simulink model "shahidspwmthreephase"  (Simulink 7.5)
settings: Solver=ode45  StartTime=0.0  StopTime=3  RelTol=1e-3
libraries: powerlib x11, powerlib_extras x6
settings Model: Creator=SHAHID  LastModifiedBy=SHAHID

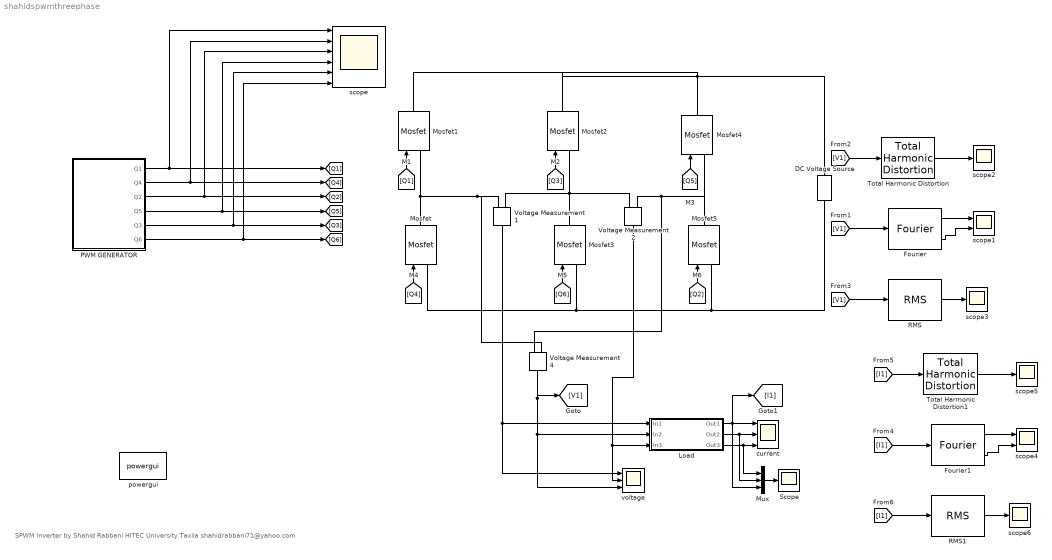
== system shahidspwmthreephase ==
  note: SPWM Inverter by Shahid Rabbani
      | HITEC University Taxila
      | shahidrabbani71@yahoo.com
  " current" : Scope  NumInputPorts=3
      settings: YMin=-0.7~-0.8~-0.7  YMax=0.8~0.7~0.7
  DC Voltage Source : powerlib/Electrical Sources/DC Voltage Source  DialogController=POWERSYS.PowerSysDialog  SystemSampleTime=-1  Amplitude=400  Measurements=Voltage
  Fourier : powerlib_extras/Measurements/Fourier  DialogController=POWERSYS.PowerSysDialog  SystemSampleTime=-1  f1=50  n=3
  Fourier1 : powerlib_extras/Measurements/Fourier  DialogController=POWERSYS.PowerSysDialog  SystemSampleTime=-1  f1=50  n=3
  Load : Subsystem
  Mosfet{,1..5} (6 alike) : powerlib/Power Electronics/Mosfet  DialogController=POWERSYS.PowerSysDialog  SystemSampleTime=-1  Ron=0.01  Lon=0  Rd=0.01  Vfd=0  IC=0  Rs=1e5  Cs=inf  Measurements=off
  Mux : Mux  Inputs=3
  PWM GENERATOR : Subsystem
  RMS : powerlib_extras/Measurements/RMS  DialogController=POWERSYS.PowerSysDialog  SystemSampleTime=-1  f1=50
  RMS1 : powerlib_extras/Measurements/RMS  DialogController=POWERSYS.PowerSysDialog  SystemSampleTime=-1  f1=50
  Scope : Scope
      settings: YMin=-1  YMax=1.2  SaveName=ScopeData2
  Total Harmonic Distortion : powerlib_extras/Measurements/Total Harmonic Distortion  DialogController=POWERSYS.PowerSysDialog  SystemSampleTime=-1  f1=50
  Total Harmonic Distortion1 : powerlib_extras/Measurements/Total Harmonic Distortion  DialogController=POWERSYS.PowerSysDialog  SystemSampleTime=-1  f1=50
  Voltage Measurement1 : powerlib/Measurements/Voltage Measurement  DialogController=POWERSYS.PowerSysDialog  SystemSampleTime=-1  PhasorSimulation=off  OutputType=Complex  PSBequivalent=0
  Voltage Measurement2 : powerlib/Measurements/Voltage Measurement  DialogController=POWERSYS.PowerSysDialog  SystemSampleTime=-1  PhasorSimulation=off  OutputType=Complex  PSBequivalent=0
  Voltage Measurement4 : powerlib/Measurements/Voltage Measurement  DialogController=POWERSYS.PowerSysDialog  SystemSampleTime=-1  PhasorSimulation=off  OutputType=Complex  PSBequivalent=0
  powergui : powerlib/powergui  Priority=1  SystemSampleTime=-1  SimulationMode=Continuous  SampleTime=50e-6  frequency=60  SPID=off  DisableSnubberDevices=off  DisableRonSwitches=off  DisableVfSwitches=off  SwTol=0  Interpol=off  frequencyindice=0  echomessages=off  HookPort=off  DisplayEquations=off  FunctionMessages=off  EnableUseOfTLC=off  x0status=blocks  RestoreLinks=warning  ResistiveCurrentMeasurement=off  Ylog=off  Xlog=on  ShowGrid=off  save=off  variable=ZData  ZoomFFT=off  StartTime=0.0  cycles=1  DisplayStyle=1  FreqAxis=off  MaxFrequency=1000  frequencyindicesteady=1  display=off  methode=off
  scope : Scope  NumInputPorts=6
      settings: YMin=0~0~0~0~0~0  YMax=1~1~1~1~1~1
  scope1 : Scope  NumInputPorts=2
      settings: YMin=-0.8~-150  YMax=0.8~150  SaveName=ScopeData3
  scope{2..3,5..6} (4 alike) : Scope
      scope2 settings: YMin=-1  YMax=1  SaveName=ScopeData4
      scope3 settings: YMin=72.241  YMax=72.241  SaveName=ScopeData5
      scope5 settings: YMin=-1  YMax=1  SaveName=ScopeData8
      scope6 settings: YMin=68.629  YMax=75.853  SaveName=ScopeData9
  scope4 : Scope  NumInputPorts=2
      settings: YMin=-0.8~-150  YMax=0.8~150  SaveName=ScopeData7
  "voltage " : Scope  NumInputPorts=3
      settings: YMin=-150~-1~-5  YMax=150~1~5  SaveName=ScopeData6
  wires:
  [Q3] -> Mosfet2/1
  [Q1] -> Mosfet1/1
  Fourier/1 -> scope1/1
  Fourier/2 -> scope1/2
  [V1] -> Fourier/1
  Total Harmonic Distortion/1 -> scope2/1
  [V1] -> Total Harmonic Distortion/1
  RMS/1 -> scope3/1
  [V1] -> RMS/1
  [Q5] -> Mosfet4/1
  [Q4] -> Mosfet/1
  [Q6] -> Mosfet3/1
  [Q2] -> Mosfet5/1
  PWM GENERATOR/1(Q1) -> [Q1], scope/1
  PWM GENERATOR/2(Q4) -> [Q4], scope/2
  PWM GENERATOR/3(Q2) -> [Q2], scope/3
  PWM GENERATOR/4(Q5) -> [Q5], scope/4
  PWM GENERATOR/5(Q3) -> [Q3], scope/5
  PWM GENERATOR/6(Q6) -> [Q6], scope/6
  Voltage Measurement1/1 -> "voltage "/1, Load/1(In1)
  Voltage Measurement2/1 -> "voltage "/2, Load/3(In3)
  Voltage Measurement4/1 -> "voltage "/3, Load/2(In2), [V1]
  Load/1(Out1) -> " current"/1, Mux/3, [I1]
  Load/2(Out2) -> " current"/2, Mux/2
  Load/3(Out3) -> " current"/3, Mux/1
  Mux/1 -> Scope/1
  Fourier1/1 -> scope4/1
  Fourier1/2 -> scope4/2
  [I1] -> Fourier1/1
  Total Harmonic Distortion1/1 -> scope5/1
  [I1] -> Total Harmonic Distortion1/1
  RMS1/1 -> scope6/1
  [I1] -> RMS1/1
  connections:
  Mosfet1/RConn1 -- Mosfet2/RConn1 -- Mosfet4/RConn1 -- DC Voltage Source/RConn1
  Mosfet3/RConn1 -- Mosfet2/LConn1 -- Voltage Measurement1/LConn2 -- Voltage Measurement2/LConn1
  Voltage Measurement1/LConn1 -- Mosfet1/LConn1 -- Mosfet/RConn1 -- Voltage Measurement4/LConn2
  Mosfet5/LConn1 -- Mosfet3/LConn1 -- Mosfet/LConn1 -- DC Voltage Source/LConn1
  Mosfet5/RConn1 -- Mosfet4/LConn1 -- Voltage Measurement2/LConn2 -- Voltage Measurement4/LConn1

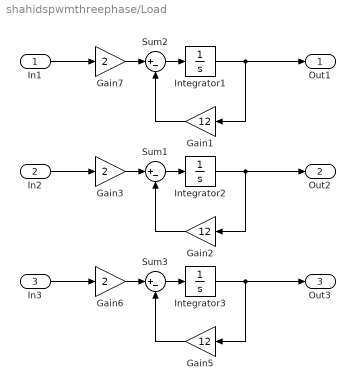
== system shahidspwmthreephase/Load ==
  In1 : Inport  OutDataType=fixdt(1, 16)  OutScaling=2^0
  In2 : Inport  Port=2  OutDataType=fixdt(1, 16)  OutScaling=2^0
  In3 : Inport  Port=3  OutDataType=fixdt(1, 16)  OutScaling=2^0
  Gain1 : Gain  Gain=12  ParameterDataType=fixdt(1, 16)  ParameterScaling=2^0  OutDataType=fixdt(1, 16)  OutScaling=2^0
  Gain2 : Gain  Gain=12  ParameterDataType=fixdt(1, 16)  ParameterScaling=2^0  OutDataType=fixdt(1, 16)  OutScaling=2^0
  Gain3 : Gain  Gain=2  ParameterDataType=fixdt(1, 16)  ParameterScaling=2^0  OutDataType=fixdt(1, 16)  OutScaling=2^0
  Gain5 : Gain  Gain=12  ParameterDataType=fixdt(1, 16)  ParameterScaling=2^0  OutDataType=fixdt(1, 16)  OutScaling=2^0
  Gain6 : Gain  Gain=2  ParameterDataType=fixdt(1, 16)  ParameterScaling=2^0  OutDataType=fixdt(1, 16)  OutScaling=2^0
  Gain7 : Gain  Gain=2  ParameterDataType=fixdt(1, 16)  ParameterScaling=2^0  OutDataType=fixdt(1, 16)  OutScaling=2^0
  Integrator1 : Integrator
  Integrator2 : Integrator
  Integrator3 : Integrator
  Sum1 : Sum  Inputs=|+-  OutDataType=fixdt(1, 16)  OutScaling=2^0
  Sum2 : Sum  Inputs=|+-  OutDataType=fixdt(1, 16)  OutScaling=2^0
  Sum3 : Sum  Inputs=|+-  OutDataType=fixdt(1, 16)  OutScaling=2^0
  Out1 : Outport  OutDataType=fixdt(1, 16)  OutScaling=2^0
  Out2 : Outport  Port=2  OutDataType=fixdt(1, 16)  OutScaling=2^0
  Out3 : Outport  Port=3  OutDataType=fixdt(1, 16)  OutScaling=2^0
  wires:
  Integrator1/1 -> Gain1/1, Out1/1
  Gain7/1 -> Sum2/1
  Sum2/1 -> Integrator1/1
  Gain1/1 -> Sum2/2
  In1/1 -> Gain7/1
  Integrator2/1 -> Gain2/1, Out2/1
  Gain3/1 -> Sum1/1
  Sum1/1 -> Integrator2/1
  Gain2/1 -> Sum1/2
  In2/1 -> Gain3/1
  Integrator3/1 -> Gain5/1, Out3/1
  Gain6/1 -> Sum3/1
  Sum3/1 -> Integrator3/1
  Gain5/1 -> Sum3/2
  In3/1 -> Gain6/1

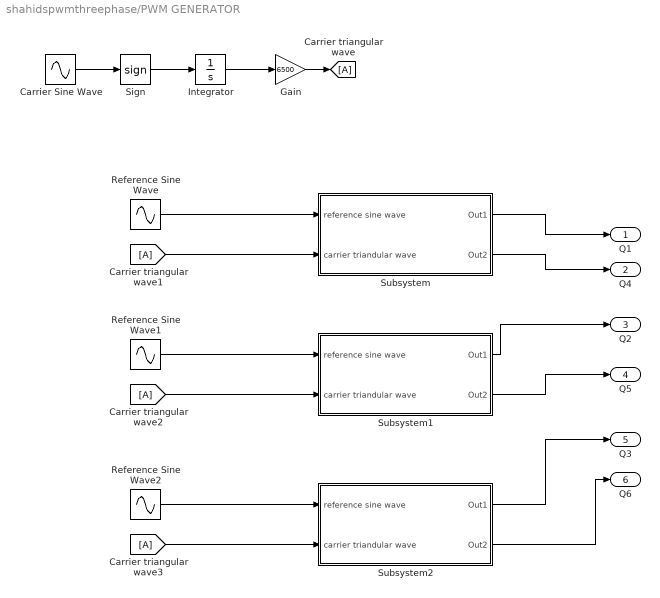
== system shahidspwmthreephase/PWM GENERATOR ==
  Carrier Sine Wave : Sin  Amplitude=1  Bias=0  Frequency=2*pi*3000  Phase=0  Samples=10  SampleTime=0  Offset=0
  Gain : Gain  Gain=6500  ParameterDataType=fixdt(1, 16)  ParameterScaling=2^0  OutDataType=fixdt(1, 16)  OutScaling=2^0
  Integrator : Integrator
  Reference Sine Wave : Sin  Amplitude=1  Bias=0  Frequency=2*pi*50  Phase=0  Samples=10  SampleTime=0  Offset=0
  Reference Sine Wave1 : Sin  Amplitude=1  Bias=0  Frequency=2*pi*50  Phase=-pi/3  Samples=10  SampleTime=0  Offset=0
  Reference Sine Wave2 : Sin  Amplitude=1  Bias=0  Frequency=2*pi*50  Phase=-2*pi/3  Samples=10  SampleTime=0  Offset=0
  Sign : Signum
  Subsystem : Subsystem
  Subsystem1 : Subsystem
  Subsystem2 : Subsystem
  Q1 : Outport  OutDataType=fixdt(1, 16)  OutScaling=2^0
  Q4 : Outport  Port=2  OutDataType=fixdt(1, 16)  OutScaling=2^0
  Q2 : Outport  Port=3  OutDataType=fixdt(1, 16)  OutScaling=2^0
  Q5 : Outport  Port=4  OutDataType=fixdt(1, 16)  OutScaling=2^0
  Q3 : Outport  Port=5  OutDataType=fixdt(1, 16)  OutScaling=2^0
  Q6 : Outport  Port=6  OutDataType=fixdt(1, 16)  OutScaling=2^0
  wires:
  Carrier Sine Wave/1 -> Sign/1
  Sign/1 -> Integrator/1
  Integrator/1 -> Gain/1
  Gain/1 -> [A]
  Reference Sine Wave/1 -> Subsystem/1(reference sine wave)
  Reference Sine Wave1/1 -> Subsystem1/1(reference sine wave)
  Reference Sine Wave2/1 -> Subsystem2/1(reference sine wave)
  [A] -> Subsystem/2(carrier triandular wave)
  [A] -> Subsystem2/2(carrier triandular wave)
  [A] -> Subsystem1/2(carrier triandular wave)
  Subsystem/1(Out1) -> Q1/1
  Subsystem/2(Out2) -> Q4/1
  Subsystem1/1(Out1) -> Q2/1
  Subsystem1/2(Out2) -> Q5/1
  Subsystem2/1(Out1) -> Q3/1
  Subsystem2/2(Out2) -> Q6/1

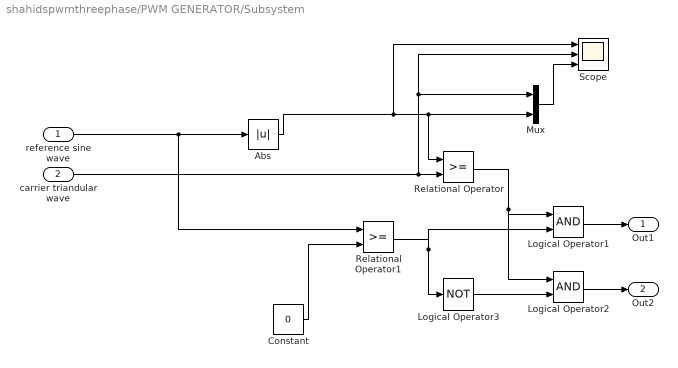
== system shahidspwmthreephase/PWM GENERATOR/Subsystem ==
  reference sine wave : Inport  OutDataType=fixdt(1, 16)  OutScaling=2^0
  carrier triandular wave : Inport  Port=2  OutDataType=fixdt(1, 16)  OutScaling=2^0
  Abs : Abs  OutDataType=fixdt(1, 16)  OutScaling=2^0
  Constant : Constant  Value=0  OutDataType=fixdt(1, 16)  OutScaling=2^0
  Logical Operator1 : Logic  AllPortsSameDT=off  OutDataTypeMode=boolean  LogicDataType=fixdt(0, 8)  OutDataTypeStr=boolean
  Logical Operator2 : Logic  AllPortsSameDT=off  OutDataTypeMode=boolean  LogicDataType=fixdt(0, 8)  OutDataTypeStr=boolean
  Logical Operator3 : Logic  Operator=NOT  AllPortsSameDT=off  OutDataTypeMode=boolean  LogicDataType=fixdt(0, 8)  OutDataTypeStr=boolean
  Mux : Mux  Inputs=2
  Relational Operator : RelationalOperator  LogicDataType=fixdt(1,16)  InputSameDT=on
  Relational Operator1 : RelationalOperator  LogicDataType=fixdt(1,16)  InputSameDT=on
  Scope : Scope  NumInputPorts=3
      settings: TickLabels=on  TimeRange=3  YMin=5.55112e-017~-0.1~-0.1  YMax=1~1.1~1.1  SaveName=ScopeData10
  Out1 : Outport  OutDataType=fixdt(1, 16)  OutScaling=2^0
  Out2 : Outport  Port=2  OutDataType=fixdt(1, 16)  OutScaling=2^0
  wires:
  Abs/1 -> Scope/1, Relational Operator/1, Mux/2
  Logical Operator3/1 -> Logical Operator2/2
  Relational Operator/1 -> Logical Operator1/1, Logical Operator2/1
  Constant/1 -> Relational Operator1/2
  Relational Operator1/1 -> Logical Operator3/1, Logical Operator1/2
  Logical Operator1/1 -> Out1/1
  Logical Operator2/1 -> Out2/1
  Mux/1 -> Scope/3
  reference sine wave/1 -> Abs/1, Relational Operator1/1
  carrier triandular wave/1 -> Relational Operator/2, Scope/2, Mux/1

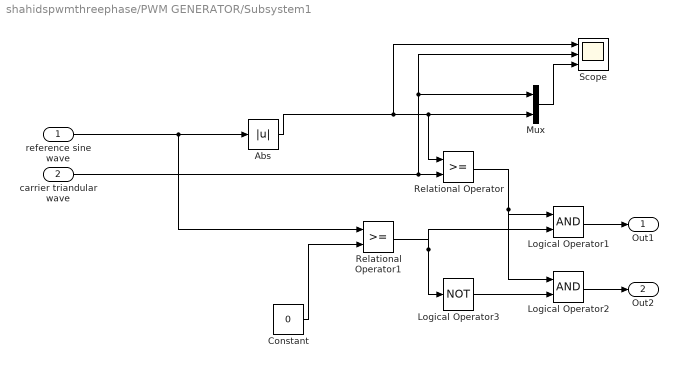
== system shahidspwmthreephase/PWM GENERATOR/Subsystem1 ==
  reference sine wave : Inport  OutDataType=fixdt(1, 16)  OutScaling=2^0
  carrier triandular wave : Inport  Port=2  OutDataType=fixdt(1, 16)  OutScaling=2^0
  Abs : Abs  OutDataType=fixdt(1, 16)  OutScaling=2^0
  Constant : Constant  Value=0  OutDataType=fixdt(1, 16)  OutScaling=2^0
  Logical Operator1 : Logic  AllPortsSameDT=off  OutDataTypeMode=boolean  LogicDataType=fixdt(0, 8)  OutDataTypeStr=boolean
  Logical Operator2 : Logic  AllPortsSameDT=off  OutDataTypeMode=boolean  LogicDataType=fixdt(0, 8)  OutDataTypeStr=boolean
  Logical Operator3 : Logic  Operator=NOT  AllPortsSameDT=off  OutDataTypeMode=boolean  LogicDataType=fixdt(0, 8)  OutDataTypeStr=boolean
  Mux : Mux  Inputs=2
  Relational Operator : RelationalOperator  LogicDataType=fixdt(1,16)  InputSameDT=on
  Relational Operator1 : RelationalOperator  LogicDataType=fixdt(1,16)  InputSameDT=on
  Scope : Scope  NumInputPorts=3
      settings: TickLabels=on  TimeRange=3  YMin=5.55112e-017~-0.1~-0.1  YMax=1~1.1~1.1  SaveName=ScopeData10
  Out1 : Outport  OutDataType=fixdt(1, 16)  OutScaling=2^0
  Out2 : Outport  Port=2  OutDataType=fixdt(1, 16)  OutScaling=2^0
  wires:
  Abs/1 -> Scope/1, Relational Operator/1, Mux/2
  Logical Operator3/1 -> Logical Operator2/2
  Relational Operator/1 -> Logical Operator1/1, Logical Operator2/1
  Constant/1 -> Relational Operator1/2
  Relational Operator1/1 -> Logical Operator3/1, Logical Operator1/2
  Logical Operator1/1 -> Out1/1
  Logical Operator2/1 -> Out2/1
  Mux/1 -> Scope/3
  reference sine wave/1 -> Abs/1, Relational Operator1/1
  carrier triandular wave/1 -> Relational Operator/2, Scope/2, Mux/1

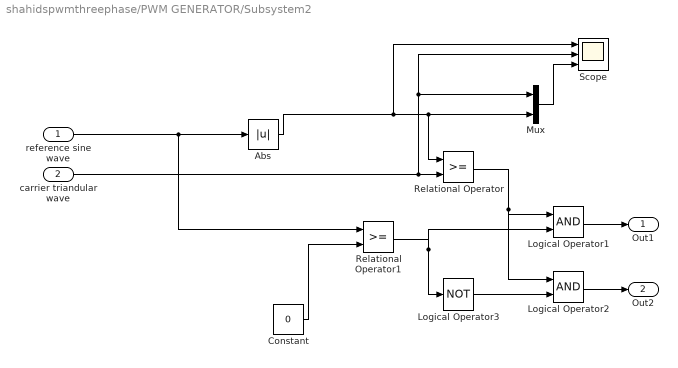
== system shahidspwmthreephase/PWM GENERATOR/Subsystem2 ==
  reference sine wave : Inport  OutDataType=fixdt(1, 16)  OutScaling=2^0
  carrier triandular wave : Inport  Port=2  OutDataType=fixdt(1, 16)  OutScaling=2^0
  Abs : Abs  OutDataType=fixdt(1, 16)  OutScaling=2^0
  Constant : Constant  Value=0  OutDataType=fixdt(1, 16)  OutScaling=2^0
  Logical Operator1 : Logic  AllPortsSameDT=off  OutDataTypeMode=boolean  LogicDataType=fixdt(0, 8)  OutDataTypeStr=boolean
  Logical Operator2 : Logic  AllPortsSameDT=off  OutDataTypeMode=boolean  LogicDataType=fixdt(0, 8)  OutDataTypeStr=boolean
  Logical Operator3 : Logic  Operator=NOT  AllPortsSameDT=off  OutDataTypeMode=boolean  LogicDataType=fixdt(0, 8)  OutDataTypeStr=boolean
  Mux : Mux  Inputs=2
  Relational Operator : RelationalOperator  LogicDataType=fixdt(1,16)  InputSameDT=on
  Relational Operator1 : RelationalOperator  LogicDataType=fixdt(1,16)  InputSameDT=on
  Scope : Scope  NumInputPorts=3
      settings: TickLabels=on  TimeRange=3  YMin=5.55112e-017~-0.1~-0.1  YMax=1~1.1~1.1  SaveName=ScopeData10
  Out1 : Outport  OutDataType=fixdt(1, 16)  OutScaling=2^0
  Out2 : Outport  Port=2  OutDataType=fixdt(1, 16)  OutScaling=2^0
  wires:
  Abs/1 -> Scope/1, Relational Operator/1, Mux/2
  Logical Operator3/1 -> Logical Operator2/2
  Relational Operator/1 -> Logical Operator1/1, Logical Operator2/1
  Constant/1 -> Relational Operator1/2
  Relational Operator1/1 -> Logical Operator3/1, Logical Operator1/2
  Logical Operator1/1 -> Out1/1
  Logical Operator2/1 -> Out2/1
  Mux/1 -> Scope/3
  reference sine wave/1 -> Abs/1, Relational Operator1/1
  carrier triandular wave/1 -> Relational Operator/2, Scope/2, Mux/1
